simulink model "robot_model"  (R2024b)
settings: Solver=VariableStepAuto  StartTime=0.0  StopTime=10.0  RelTol=1e-3
values from neighbouring files (symbols this model uses):
  g = 9.81    [robot.m]    (also in robot_cascade.m; robot_linear.m; robot_lqr.m)
  Jm = J - Jp    (= -0.00769717)    [robot.m]
  Jp = m*l^2    (= 0.0077625)    [robot.m]    (also in robot_cascade.m = 6.533e-05; robot_linear.m = 6.533e-05; robot_lqr.m = 6.533e-05)
  Jp_delta = 9.0372e-5    (= 9.0372e-05)    [robot.m]
  Jw = 1/2*Mw*R^2    (= 4e-07)    [robot.m]    (also in robot_cascade.m = 1e-08; robot_linear.m; robot_lqr.m = 1e-08)
  Km = 16.129/1000    (= 0.016129)    [robot.m]    (also in robot_cascade.m = 16.1290322581; robot_linear.m = 0.212207; robot_lqr.m = 0.212207)
  l = 0.15    [robot.m]    (also in robot_cascade.m = 0.08; robot_linear.m = 0.08)
  l_axel = 0.2359    [robot.m]    (also in robot_cascade.m; robot_linear.m; robot_lqr.m)
  M = 1.285    [robot.m]    (also in robot_cascade.m = 1.18; robot_linear.m = 1.18; robot_lqr.m = 1.18)
  m = mtot-M    (= 0.345)    [robot.m]    (also in robot_cascade.m = 0.33; robot_linear.m = 0.33; robot_lqr.m = 0.33)
  Mw = 0.0005    [robot.m]    (also in robot_linear.m)
  n = 18.75    [robot.m]    (also in robot_cascade.m; robot_linear.m; robot_lqr.m)
  R = 1    [invgui.m]    (also in robot.m = 0.04; robot_lqr.m = 200)
libraries: cstblocks x4, slpidlib x3
settings Model: Creator=cosr3  LastModifiedBy=cosr3

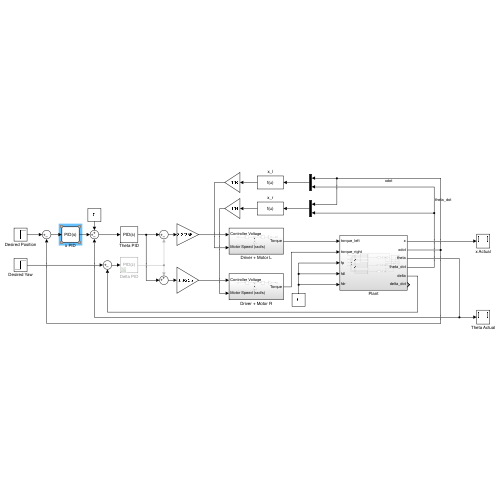
[thumbnail: Simulink's stored preview of the top-level diagram]
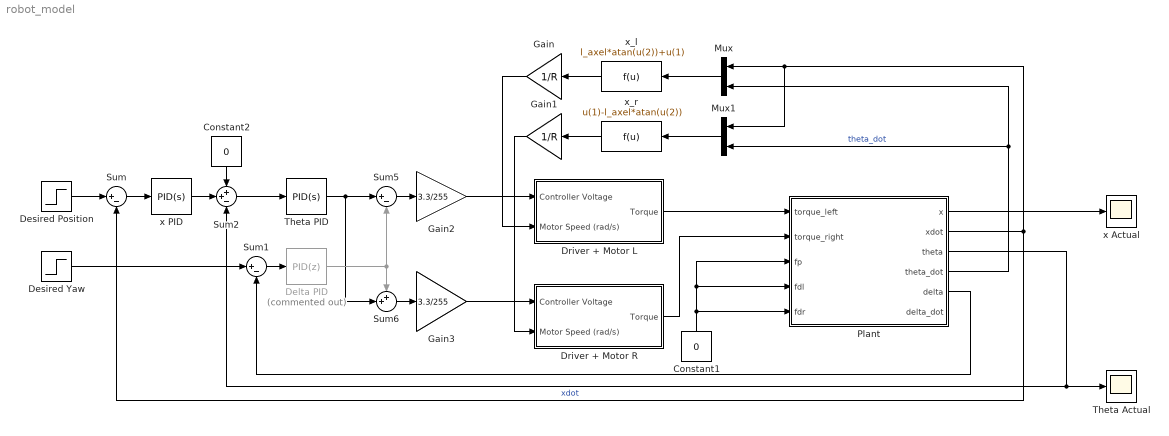
== system robot_model ==
  Constant1 : Constant  Value=0
  Constant2 : Constant  Value=0
  Delta PID : slpidlib/PID Controller  Commented=on  Controller=PID  Form=Parallel  TimeDomain=Discrete-time  UseExternalTs=off  SampleTime=1/550  IntegratorMethod=Forward Euler  FilterMethod=Forward Euler  ControllerParametersSource=internal  P=-0.0147063328753403  I=-0.00136714449093344  UseKiTs=off  D=-0.0214383336905415  UseExternalDerivativeSource=off  N=1448.28246069918  UseFilter=on  TunerSelectOption=Transfer Function Based (PID Tuner App)  InitialConditionSource=internal  InitialConditionForIntegrator=0  InitialConditionForFilter=0  DifferentiatorICPrevScaledInput=0  ExternalReset=none  TrackingMode=off  Kt=1  LimitOutput=off  SatLimitsSource=internal  UpperSaturationLimit=inf  LowerSaturationLimit=-inf  LinearizeAsGain=off  AntiWindupMode=none  Kb=1  LimitIntegrator=off  UpperIntegratorSaturationLimit=inf  LowerIntegratorSaturationLimit=-inf  POutMin=[]  POutMax=[]  IOutMin=[]  IOutMax=[]  DOutMin=[]  DOutMax=[]  NOutMin=[]  NOutMax=[]  SumOutMin=[]  SumOutMax=[]  SaturationOutMin=[]  SaturationOutMax=[]  PParamMin=[]  PParamMax=[]  IParamMin=[]  IParamMax=[]  DParamMin=[]  DParamMax=[]  NParamMin=[]  NParamMax=[]  KbParamMin=[]  KbParamMax=[]  KtParamMin=[]  KtParamMax=[]  KbOutMin=[]  KbOutMax=[]  KtOutMin=[]  KtOutMax=[]  IntegratorOutMin=[]  IntegratorOutMax=[]  FilterOutMin=[]  FilterOutMax=[]  SumI1OutMin=[]  SumI1OutMax=[]  SumI2OutMin=[]  SumI2OutMax=[]  SumI3OutMin=[]  SumI3OutMax=[]  SumI4OutMin=[]  SumI4OutMax=[]  SumDOutMin=[]  SumDOutMax=[]  DifferentiatorOutMin=[]  DifferentiatorOutMax=[]  FilterDiffOutCoefMin=[]  FilterDiffOutCoefMax=[]  ReciprocalOutMin=[]  ReciprocalOutMax=[]  SumDenOutMin=[]  SumDenOutMax=[]  SumNumOutMin=[]  SumNumOutMax=[]  DivideOutMin=[]  DivideOutMax=[]  UdiffTsProdOutMin=[]  UdiffTsProdOutMax=[]  NTsProdOutMin=[]  NTsProdOutMax=[]  UintegralTsProdOutMin=[]  UintegralTsProdOutMax=[]  UngainTsProdOutMin=[]  UngainTsProdOutMax=[]  ClampingZeroOutDataTypeStr=Inherit: Inherit via back propagation  ClampingZeroOutMin=[]  ClampingZeroOutMax=[]  FilterDenConstantOutDataTypeStr=Inherit: Inherit via back propagation  FilterDenConstantOutMin=[]  FilterDenConstantOutMax=[]  PCopyOutDataTypeStr=Inherit: Inherit via back propagation  PCopyOutMin=[]  PCopyOutMax=[]  NCopyOutDataTypeStr=Inherit: Inherit via back propagation  NCopyOutMin=[]  NCopyOutMax=[]  IntegratorContinuousStateAttributes=''  IntegratorStateMustResolveToSignalObject=off  IntegratorRTWStateStorageClass=Auto  FilterContinuousStateAttributes=''  FilterStateMustResolveToSignalObject=off  FilterRTWStateStorageClass=Auto  ParallelPVariant=InternalParameters  IdealPVariant=Disabled  IVariant=InternalParameters  DVariant=InternalParameters  IntegratorVariant=Discrete  SatVariant=Disabled  AWVariant=Passthrough  PCopyVariant=Disabled  TRVariant=Disabled  FdbkBlocksVariant=Forward  IdealPFdbkVariant=Disabled  SatFdbkVariant=Disabled  DerivativeFilterVariant=ForwardEulerFilter  NVariant=InternalParameters  NCopyVariant=Disabled  FilterICVariant=InternalICsFilter  IntegratorICVariant=InternalICs  ExternalResetVariant=Disabled  TRSumVariant=Passthrough  SumFdbkVariant=Disabled  SumVariant=Sum_PID  TsampFilterVariant=InternalTs  TsampNgainVariant=Passthrough  TsampIntegralVariant=Disabled_SignalSpec  ExternalSaturationOutDataTypeStr=Inherit: Same as second input  DerivativeSourceVariant=ErrorSignal  PreIntVariant=InternalPreInt
      settings: LibrarySourceBlock=simulink/Discrete/Discrete PID Controller
  Desired Position : Step  SampleTime=0
  Desired Yaw : Step  SampleTime=0
  Driver + Motor L : Subsystem
  Driver + Motor R : Subsystem
  Gain : Gain  Gain=1/R
  Gain1 : Gain  Gain=1/R
  Gain2 : Gain  Gain=3.3/255
  Gain3 : Gain  Gain=3.3/255
  Mux : Mux  Inputs=2
  Mux1 : Mux  Inputs=2
  Plant : Subsystem
  Sum : Sum  Inputs=|+-
  Sum1 : Sum  Inputs=|+-
  Sum2 : Sum  Inputs=++-
  Sum5 : Sum  Inputs=|+-
  Sum6 : Sum  Inputs=++|
  Theta Actual : Scope
  Theta PID : slpidlib/PID Controller  Controller=PID  Form=Ideal  TimeDomain=Continuous-time  UseExternalTs=off  SampleTime=-1  IntegratorMethod=Forward Euler  FilterMethod=Forward Euler  ControllerParametersSource=internal  P=5792.95362494013  I=5.30299616336918  UseKiTs=on  D=0.0216080818218296  UseExternalDerivativeSource=off  N=24990.0250158816  UseFilter=on  TunerSelectOption=Transfer Function Based (PID Tuner App)  InitialConditionSource=internal  InitialConditionForIntegrator=0  InitialConditionForFilter=0  DifferentiatorICPrevScaledInput=0  ExternalReset=none  TrackingMode=off  Kt=1  LimitOutput=off  SatLimitsSource=internal  UpperSaturationLimit=inf  LowerSaturationLimit=-inf  LinearizeAsGain=off  AntiWindupMode=none  Kb=1  LimitIntegrator=off  UpperIntegratorSaturationLimit=inf  LowerIntegratorSaturationLimit=-inf  POutMin=[]  POutMax=[]  IOutMin=[]  IOutMax=[]  DOutMin=[]  DOutMax=[]  NOutMin=[]  NOutMax=[]  SumOutMin=[]  SumOutMax=[]  SaturationOutMin=[]  SaturationOutMax=[]  PParamMin=[]  PParamMax=[]  IParamMin=[]  IParamMax=[]  DParamMin=[]  DParamMax=[]  NParamMin=[]  NParamMax=[]  KbParamMin=[]  KbParamMax=[]  KtParamMin=[]  KtParamMax=[]  KbOutMin=[]  KbOutMax=[]  KtOutMin=[]  KtOutMax=[]  IntegratorOutMin=[]  IntegratorOutMax=[]  FilterOutMin=[]  FilterOutMax=[]  SumI1OutMin=[]  SumI1OutMax=[]  SumI2OutMin=[]  SumI2OutMax=[]  SumI3OutMin=[]  SumI3OutMax=[]  SumI4OutMin=[]  SumI4OutMax=[]  SumDOutMin=[]  SumDOutMax=[]  DifferentiatorOutMin=[]  DifferentiatorOutMax=[]  FilterDiffOutCoefMin=[]  FilterDiffOutCoefMax=[]  ReciprocalOutMin=[]  ReciprocalOutMax=[]  SumDenOutMin=[]  SumDenOutMax=[]  SumNumOutMin=[]  SumNumOutMax=[]  DivideOutMin=[]  DivideOutMax=[]  UdiffTsProdOutMin=[]  UdiffTsProdOutMax=[]  NTsProdOutMin=[]  NTsProdOutMax=[]  UintegralTsProdOutMin=[]  UintegralTsProdOutMax=[]  UngainTsProdOutMin=[]  UngainTsProdOutMax=[]  ClampingZeroOutDataTypeStr=Inherit: Inherit via back propagation  ClampingZeroOutMin=[]  ClampingZeroOutMax=[]  FilterDenConstantOutDataTypeStr=Inherit: Inherit via back propagation  FilterDenConstantOutMin=[]  FilterDenConstantOutMax=[]  PCopyOutDataTypeStr=Inherit: Inherit via back propagation  PCopyOutMin=[]  PCopyOutMax=[]  NCopyOutDataTypeStr=Inherit: Inherit via back propagation  NCopyOutMin=[]  NCopyOutMax=[]  IntegratorContinuousStateAttributes=''  IntegratorStateMustResolveToSignalObject=off  IntegratorRTWStateStorageClass=Auto  FilterContinuousStateAttributes=''  FilterStateMustResolveToSignalObject=off  FilterRTWStateStorageClass=Auto  ParallelPVariant=Passthrough  IdealPVariant=InternalParameters  IVariant=InternalParameters  DVariant=InternalParameters  IntegratorVariant=Continuous  SatVariant=Disabled  AWVariant=Passthrough  PCopyVariant=Disabled  TRVariant=Disabled  FdbkBlocksVariant=Forward  IdealPFdbkVariant=Disabled  SatFdbkVariant=Disabled  DerivativeFilterVariant=ContFilter  NVariant=InternalParameters  NCopyVariant=Disabled  FilterICVariant=InternalICsFilter  IntegratorICVariant=InternalICs  ExternalResetVariant=Disabled  TRSumVariant=Passthrough  SumFdbkVariant=Disabled  SumVariant=Sum_PID  TsampFilterVariant=InternalTs  TsampNgainVariant=Passthrough  TsampIntegralVariant=Disabled_SignalSpec  ExternalSaturationOutDataTypeStr=Inherit: Same as second input  DerivativeSourceVariant=ErrorSignal  PreIntVariant=InternalPreInt
      settings: LibrarySourceBlock=simulink/Discrete/Discrete PID Controller
  x Actual : Scope
  x PID : slpidlib/PID Controller  Controller=PID  Form=Parallel  TimeDomain=Continuous-time  UseExternalTs=off  SampleTime=-1  IntegratorMethod=Forward Euler  FilterMethod=Forward Euler  ControllerParametersSource=internal  P=-0.0628292562730309  I=-0.000431329975665461  UseKiTs=on  D=-2.03345781963945  UseExternalDerivativeSource=off  N=134.483020197825  UseFilter=on  TunerSelectOption=Transfer Function Based (PID Tuner App)  InitialConditionSource=internal  InitialConditionForIntegrator=0  InitialConditionForFilter=0  DifferentiatorICPrevScaledInput=0  ExternalReset=none  TrackingMode=off  Kt=1  LimitOutput=off  SatLimitsSource=internal  UpperSaturationLimit=inf  LowerSaturationLimit=-inf  LinearizeAsGain=off  AntiWindupMode=none  Kb=1  LimitIntegrator=off  UpperIntegratorSaturationLimit=inf  LowerIntegratorSaturationLimit=-inf  POutMin=[]  POutMax=[]  IOutMin=[]  IOutMax=[]  DOutMin=[]  DOutMax=[]  NOutMin=[]  NOutMax=[]  SumOutMin=[]  SumOutMax=[]  SaturationOutMin=[]  SaturationOutMax=[]  PParamMin=[]  PParamMax=[]  IParamMin=[]  IParamMax=[]  DParamMin=[]  DParamMax=[]  NParamMin=[]  NParamMax=[]  KbParamMin=[]  KbParamMax=[]  KtParamMin=[]  KtParamMax=[]  KbOutMin=[]  KbOutMax=[]  KtOutMin=[]  KtOutMax=[]  IntegratorOutMin=[]  IntegratorOutMax=[]  FilterOutMin=[]  FilterOutMax=[]  SumI1OutMin=[]  SumI1OutMax=[]  SumI2OutMin=[]  SumI2OutMax=[]  SumI3OutMin=[]  SumI3OutMax=[]  SumI4OutMin=[]  SumI4OutMax=[]  SumDOutMin=[]  SumDOutMax=[]  DifferentiatorOutMin=[]  DifferentiatorOutMax=[]  FilterDiffOutCoefMin=[]  FilterDiffOutCoefMax=[]  ReciprocalOutMin=[]  ReciprocalOutMax=[]  SumDenOutMin=[]  SumDenOutMax=[]  SumNumOutMin=[]  SumNumOutMax=[]  DivideOutMin=[]  DivideOutMax=[]  UdiffTsProdOutMin=[]  UdiffTsProdOutMax=[]  NTsProdOutMin=[]  NTsProdOutMax=[]  UintegralTsProdOutMin=[]  UintegralTsProdOutMax=[]  UngainTsProdOutMin=[]  UngainTsProdOutMax=[]  ClampingZeroOutDataTypeStr=Inherit: Inherit via back propagation  ClampingZeroOutMin=[]  ClampingZeroOutMax=[]  FilterDenConstantOutDataTypeStr=Inherit: Inherit via back propagation  FilterDenConstantOutMin=[]  FilterDenConstantOutMax=[]  PCopyOutDataTypeStr=Inherit: Inherit via back propagation  PCopyOutMin=[]  PCopyOutMax=[]  NCopyOutDataTypeStr=Inherit: Inherit via back propagation  NCopyOutMin=[]  NCopyOutMax=[]  IntegratorContinuousStateAttributes=''  IntegratorStateMustResolveToSignalObject=off  IntegratorRTWStateStorageClass=Auto  FilterContinuousStateAttributes=''  FilterStateMustResolveToSignalObject=off  FilterRTWStateStorageClass=Auto  ParallelPVariant=InternalParameters  IdealPVariant=Disabled  IVariant=InternalParameters  DVariant=InternalParameters  IntegratorVariant=Continuous  SatVariant=Disabled  AWVariant=Passthrough  PCopyVariant=Disabled  TRVariant=Disabled  FdbkBlocksVariant=Forward  IdealPFdbkVariant=Disabled  SatFdbkVariant=Disabled  DerivativeFilterVariant=ContFilter  NVariant=InternalParameters  NCopyVariant=Disabled  FilterICVariant=InternalICsFilter  IntegratorICVariant=InternalICs  ExternalResetVariant=Disabled  TRSumVariant=Passthrough  SumFdbkVariant=Disabled  SumVariant=Sum_PID  TsampFilterVariant=InternalTs  TsampNgainVariant=Passthrough  TsampIntegralVariant=Disabled_SignalSpec  ExternalSaturationOutDataTypeStr=Inherit: Same as second input  DerivativeSourceVariant=ErrorSignal  PreIntVariant=InternalPreInt
      settings: LibrarySourceBlock=simulink/Discrete/Discrete PID Controller
  x_l : Fcn  Expr=l_axel*atan(u(2))+u(1)
  x_r : Fcn  Expr=u(1)-l_axel*atan(u(2))
  wires:
  Desired Position/1 -> Sum/1
  Sum/1 -> x PID/1
  Plant/2(xdot) -> Mux1/1, Mux/1, Sum/2  "xdot"
  Desired Yaw/1 -> Sum1/1
  Sum1/1 -> Delta PID/1
  Sum2/1 -> Theta PID/1
  Plant/3(theta) -> Theta Actual/1, Sum2/3
  Plant/1(x) -> x Actual/1
  Driver + Motor L/1(Torque) -> Plant/1(torque_left)
  Driver + Motor R/1(Torque) -> Plant/2(torque_right)
  Mux/1 -> x_l/1
  Mux1/1 -> x_r/1
  Plant/4(theta_dot) -> Mux/2, Mux1/2  "theta_dot"
  x_l/1 -> Gain/1
  x_r/1 -> Gain1/1
  Gain/1 -> Driver + Motor L/2(Motor Speed (rad/s))
  Gain1/1 -> Driver + Motor R/2(Motor Speed (rad/s))
  Theta PID/1 -> Sum5/1, Sum6/2
  Plant/5(delta) -> Sum1/2
  Constant1/1 -> Plant/4(fdl), Plant/3(fp), Plant/5(fdr)
  Gain2/1 -> Driver + Motor L/1(Controller Voltage)
  Gain3/1 -> Driver + Motor R/1(Controller Voltage)
  Constant2/1 -> Sum2/1
  Sum5/1 -> Gain2/1
  x PID/1 -> Sum2/2
  Delta PID/1 -> Sum5/2, Sum6/1
  Sum6/1 -> Gain3/1

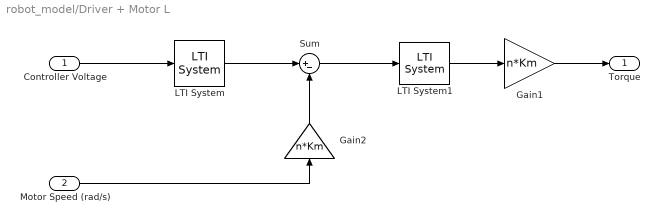
== system robot_model/Driver + Motor L ==
  Controller Voltage : Inport
  Motor Speed (rad/s) : Inport  Port=2
  Gain1 : Gain  Gain=n*Km
  Gain2 : Gain  Gain=n*Km
  LTI System : cstblocks/LTI System  sys=Ga  IC=[]  PadeOrder=0
  LTI System1 : cstblocks/LTI System  sys=Ye  IC=[]  PadeOrder=0
  Sum : Sum  Inputs=|+-
  Torque : Outport
  wires:
  Controller Voltage/1 -> LTI System/1
  LTI System1/1 -> Gain1/1
  Gain1/1 -> Torque/1
  LTI System/1 -> Sum/1
  Sum/1 -> LTI System1/1
  Gain2/1 -> Sum/2
  Motor Speed (rad/s)/1 -> Gain2/1

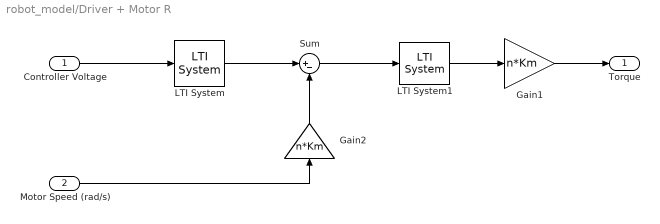
== system robot_model/Driver + Motor R ==
  Controller Voltage : Inport
  Motor Speed (rad/s) : Inport  Port=2
  Gain1 : Gain  Gain=n*Km
  Gain2 : Gain  Gain=n*Km
  LTI System : cstblocks/LTI System  sys=Ga  IC=[]  PadeOrder=0
  LTI System1 : cstblocks/LTI System  sys=Ye  IC=[]  PadeOrder=0
  Sum : Sum  Inputs=|+-
  Torque : Outport
  wires:
  Controller Voltage/1 -> LTI System/1
  LTI System1/1 -> Gain1/1
  Gain1/1 -> Torque/1
  LTI System/1 -> Sum/1
  Sum/1 -> LTI System1/1
  Gain2/1 -> Sum/2
  Motor Speed (rad/s)/1 -> Gain2/1

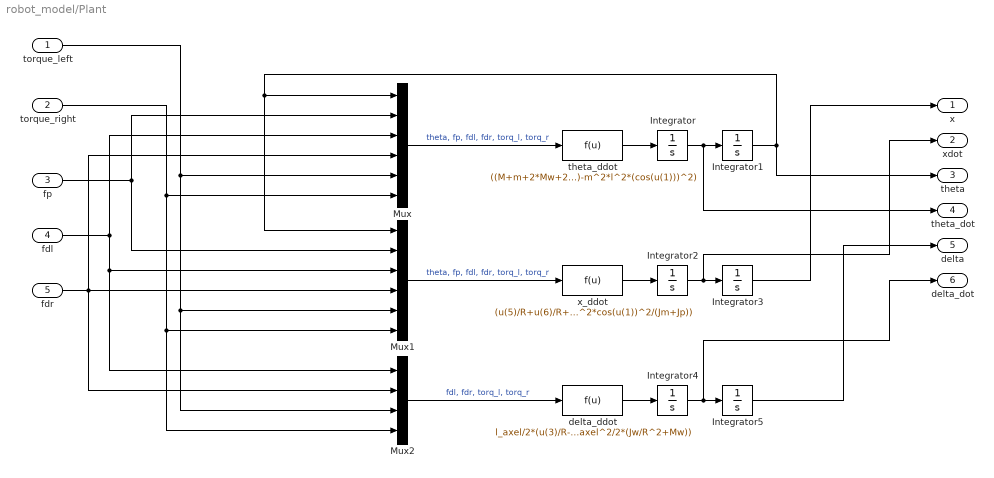
== system robot_model/Plant ==
  torque_left : Inport
  torque_right : Inport  Port=2
  fp : Inport  Port=3
  fdl : Inport  Port=4
  fdr : Inport  Port=5
  Integrator : Integrator  ContinuousStateAttributes='theta_dot'
  Integrator1 : Integrator  ContinuousStateAttributes='theta'
  Integrator{2..5} (4 alike) : Integrator
  Mux : Mux  Inputs=6
  Mux1 : Mux  Inputs=6
  Mux2 : Mux
  delta_ddot : Fcn  Expr=l_axel/2*(u(3)/R-u(2)/R+u(1)-u(2))/(Jp_delta+l_axel^2/2*(Jw/R^2+Mw))
  theta_ddot : Fcn  Expr=((M+m+2*Mw+2*Jw/R^2)*(m*g*l*sin(u(1))+u(2)*l*cos(u(1)))-m*l*cos(u(1))*(u(5)/R+u(6)/R+u(2)+u(3)+u(4)))/((Jm+Jp)*(M+m+2*Mw+2*Jw/R^2)-m^2*l^2*(cos(u(1)))^2)
  x_ddot : Fcn  Expr=(u(5)/R+u(6)/R+u(2)+u(3)+u(4)-(m*l*cos(u(1))*(m*g*l*sin(u(1))-u(2)*l*cos(u(1))))/Jm+Jp)/(M+m+2*Mw+2*Jw/R^2-m^2*l^2*cos(u(1))^2/(Jm+Jp))
  x : Outport
  xdot : Outport  Port=2
  theta : Outport  Port=3
  theta_dot : Outport  Port=4
  delta : Outport  Port=5
  delta_dot : Outport  Port=6
  wires:
  theta_ddot/1 -> Integrator/1
  Integrator/1 -> theta_dot/1, Integrator1/1
  Mux/1 -> theta_ddot/1  "theta, fp, fdl, fdr, torq_l, torq_r"
  torque_right/1 -> Mux2/4, Mux1/6, Mux/6
  fp/1 -> Mux/2, Mux1/2
  fdl/1 -> Mux/3, Mux2/1, Mux1/3
  Integrator1/1 -> theta/1, Mux/1, Mux1/1
  torque_left/1 -> Mux2/3, Mux1/5, Mux/5
  Integrator5/1 -> delta/1
  Integrator4/1 -> delta_dot/1, Integrator5/1
  Integrator2/1 -> xdot/1, Integrator3/1
  Integrator3/1 -> x/1
  Mux2/1 -> delta_ddot/1  "fdl, fdr, torq_l, torq_r"
  delta_ddot/1 -> Integrator4/1
  fdr/1 -> Mux2/2, Mux1/4, Mux/4
  x_ddot/1 -> Integrator2/1
  Mux1/1 -> x_ddot/1  "theta, fp, fdl, fdr, torq_l, torq_r"
